simulink model "ped"  (R2023a)
settings: Solver=VariableStepAuto  StartTime=0.0  StopTime=2  RelTol=1e-3
settings Model: Creator=usradmin  LastModifiedBy=harry

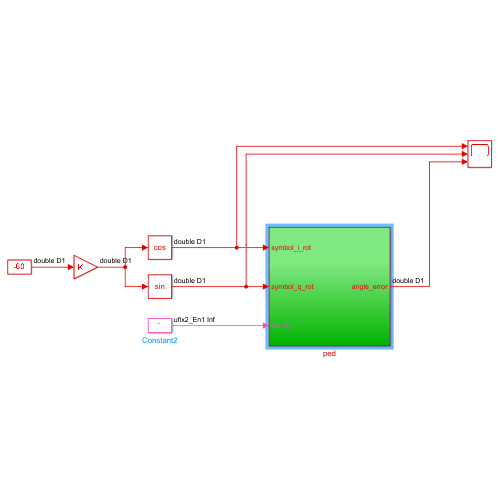
[thumbnail: Simulink's stored preview of the top-level diagram]
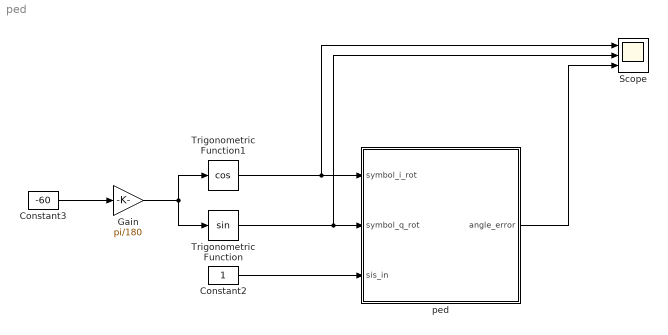
== system ped ==
  Constant2 : Constant  OutDataTypeStr=fixdt(0,2)
  Constant3 : Constant  Value=-60  OutDataTypeStr=double  SampleTime=1
  Gain : Gain  Gain=pi/180
  Scope : Scope  NumInputPorts=3
  Trigonometric Function : Trigonometry
  Trigonometric Function1 : Trigonometry  Operator=cos
  ped : Subsystem
  wires:
  Trigonometric Function/1 -> Scope/2, ped/2(symbol_q_rot)
  Trigonometric Function1/1 -> Scope/1, ped/1(symbol_i_rot)
  Constant2/1 -> ped/3(sis_in)
  Gain/1 -> Trigonometric Function1/1, Trigonometric Function/1
  Constant3/1 -> Gain/1
  ped/1(angle_error) -> Scope/3

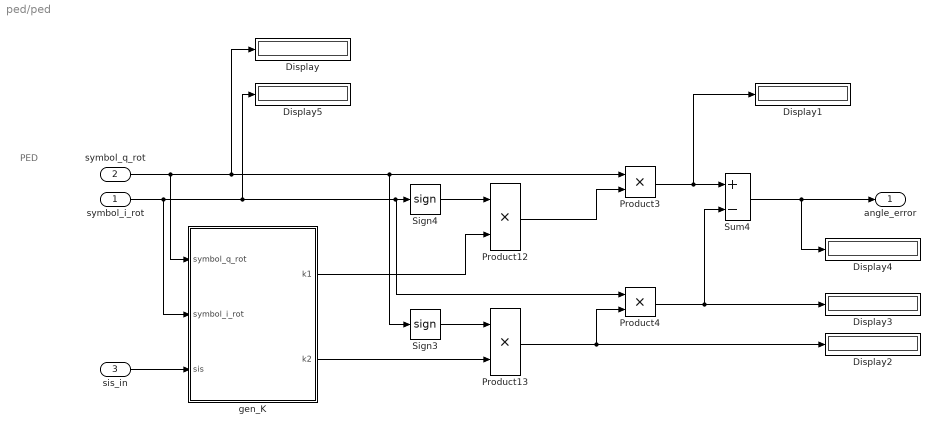
== system ped/ped ==
  note: PED
  symbol_i_rot : Inport
  symbol_q_rot : Inport  Port=2
  sis_in : Inport  Port=3
  Display{,1..5} (6 alike) : Display
  Product{3..4,12..13} (4 alike) : Product
  Sign3 : Signum
  Sign4 : Signum
  Sum4 : Sum  Inputs=+-
  gen_K : MATLAB Function  TreatAsAtomicUnit=on
  angle_error : Outport
  wires:
  gen_K/2(k2) -> Product13/2
  sis_in/1 -> gen_K/3(sis)
  Product13/1 -> Display2/1, Product4/2
  symbol_q_rot/1 -> gen_K/1(symbol_q_rot), Product3/1, Sign3/1, Display/1
  Sign4/1 -> Product12/1
  Sign3/1 -> Product13/1
  Product4/1 -> Display3/1, Sum4/2
  gen_K/1(k1) -> Product12/2
  Product12/1 -> Product3/2
  Product3/1 -> Display1/1, Sum4/1
  symbol_i_rot/1 -> gen_K/2(symbol_i_rot), Display5/1, Product4/1, Sign4/1
  Sum4/1 -> angle_error/1, Display4/1

== matlab function ped/gen_K ==
  data: symbol_q_rot input; symbol_i_rot input; k1 output; sis input; k2 output
function [k1, k2] = func_gen_K(symbol_q_rot, symbol_i_rot, sis)
% -------------------------------------------------------------------------
% Function gen_K
% -------------------------------------------------------------------------
    real_tmp = abs(symbol_i_rot);
    imag_tmp = abs(symbol_q_rot);
    
    % Determina quien es mayor la parte real o imaginaria
    if (real_tmp < imag_tmp)
        tmp = 1;
    else
        tmp = 0;
    end
    
    % calcula k1 y k2 
    if (sis == 1)
       k2 = 0;
    elseif (sis == 3 && tmp == 0)
       k2 = sqrt(2)-1;
    else
       k2 = 1;
    end

    if (sis == 3 && tmp == 1)
       k1 = sqrt(2)-1;
    else
       k1 = 1;
    end
end
% -------------------------------------------------------------------------
